simulink model "ROV_REG_SIM"  (R2014b)
settings: Solver=ode45  StartTime=0.0  StopTime=110  RelTol=1e-3
values from neighbouring files (symbols this model uses):
  ADB = 0.5    [ROV_REG.m]
  DDB = 0.8    [ROV_REG.m]
  Mass = 17    [ROV_REG.m]
  PT = [0,0,0,0,cos(ThDir(1,5:8)) ... (first row only)    [ROV_REG.m]
  rhoDB = rho/1000    (= 1)    [ROV_REG.m]
undefined symbols (not defined in the file or in its folder): magnitude
libraries: dspindex x4, vrlib x3
settings Model: Creator=Hartvik  LastModifiedBy=Hartvik

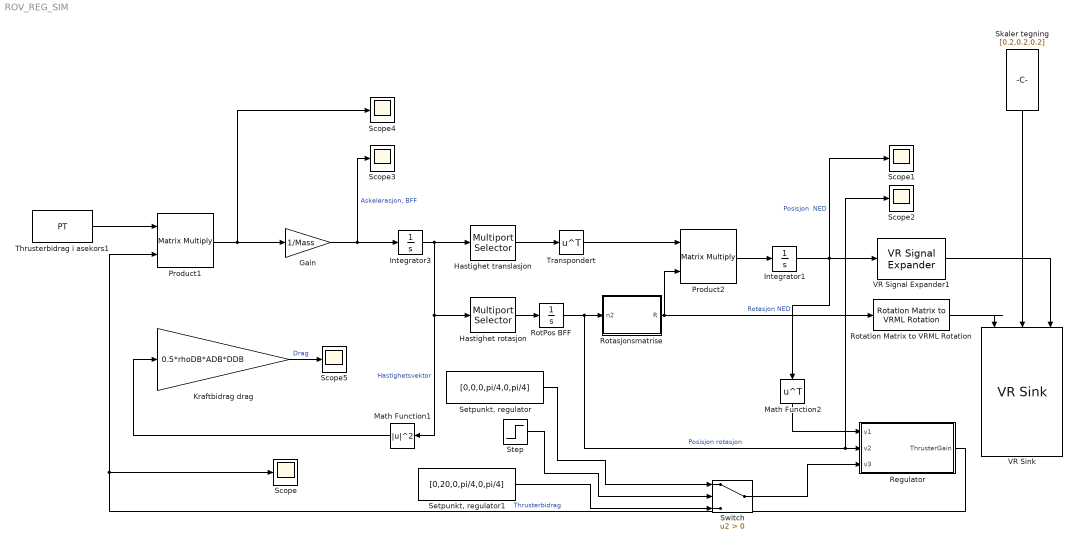
== system ROV_REG_SIM ==
  Gain : Gain  Gain=1/Mass
  Hastighet rotasjon : dspindex/Multiport Selector  rowsOrCols=Rows  idxCellArray={ 4:6}  idxErrMode=Clip Index
  Hastighet translasjon : dspindex/Multiport Selector  rowsOrCols=Rows  idxCellArray={ 1:3}  idxErrMode=Clip Index
  Integrator1 : Integrator
  Integrator3 : Integrator
  Kraftbidrag drag : Gain  Gain=0.5*rhoDB*ADB*DDB
  Math Function1 : Math  Operator=magnitude^2  SaturateOnIntegerOverflow=on
  Math Function2 : Math  Operator=transpose  SaturateOnIntegerOverflow=on
  Product1 : Product  Multiplication=Matrix(*)
  Product2 : Product  Multiplication=Matrix(*)
  Regulator : Subsystem  mask{Kd_rot=60, Kd_trans=10, Kp_rot=6, Kp_trans=1}
  RotPos BFF : Integrator
  Rotasjonsmatrise : MATLAB Function  TreatAsAtomicUnit=on
  Rotation Matrix to VRML Rotation : vrlib/Utilities/Rotation Matrix to VRML Rotation  maxzero=1e-12
  Scope{,1..5} (6 alike) : Scope
      Scope settings: YMin=-0.005  YMax=0.004
      Scope1 settings: TimeRange=37.52499999999999  YMin=0  YMax=1.4
      Scope2 settings: TimeRange=37.52499999999999  YMin=0  YMax=1.4  SaveName=ScopeData2
      Scope3 settings: YMin=-0.1  YMax=0.2  SaveName=ScopeData3
      Scope4 settings: YMin=-1e+15  YMax=8e+14  SaveName=ScopeData4
      Scope5 settings: YMin=-30  YMax=30  SaveName=ScopeData5
  "Setpunkt, regulator" : Constant  Value=[0,0,0,pi/4,0,pi/4]
  "Setpunkt, regulator1" : Constant  Value=[0,20,0,pi/4,0,pi/4]
  Skaler tegning : Constant  Value=[0.2,0.2,0.2]
  Step : Step  Time=15  Before=1  After=-1  SampleTime=0
  Switch : Switch  Criteria=u2 > Threshold
  Thrusterbidrag i asekors1 : Constant  Value=PT
  Transpondert : Math  Operator=transpose  SaturateOnIntegerOverflow=on
  VR Signal Expander1 : vrlib/VR Signal Expander  outwidth=3  outidx=[1,2,3]
  VR Sink : vrlib/VR Sink  InstantiateOnLoad=on  SampleTime=0.1  ViewEnable=on  RemoteChange=off  RemoteView=off  FieldsWritten=AUV.rotation.4.1.1.double#AUV.scale.3.1.1.double#AUV.translation.3.1.1.double  WorldFileName=D:\Dropbox\UISS-03-ROV\Elektro\Regulering\Simulink3D\AUV_emptyshell.wrl  WorldDescription=AUV_emptyshell  AutoView=off  VideoDimensions=[]  AllowVariableSize=off  FigureProperties="{'Position', 'Name', 'Viewpoint', 'CameraBound', 'CameraDirection', 'CameraPosition', 'CameraUpVector', 'ZoomFactor', 'Antialiasing', 'Headlight', 'Lighting', 'NavPanel', 'Sound', 'StatusBar', 'Stereo3D', 'Stereo3DCameraOffset', 'Stereo3DHIT', 'ToolBar', 'Textures', 'Transparency', 'Triad', 'Wireframe', 'NavZones', 'NavMode', 'NavSpeed', 'CaptureFileFormat', 'CaptureFileName', 'Record2DCompressMethod', 'Record2DCompressQuality', 'Record2D', 'Record2DFileName', 'Record2DFPS'; [5.0000000000000000e+00   9.2000000000000000e+01   5.7600000000000000e+02   3.8000000000000000e+02], 'AUV_emptyshell', 'Front', 'on', [0.0000000000000000e+00   0.0000000000000000e+00  -1.0000000000000000e+00], [0.0000000000000000e+00   0.0000000000000000e+00   0.0000000000000000e+00], [0.0000000000000000e+00   1.0000000000000000e+00   0.0000000000000000e+00], [1.0000000000000000e+00], 'on', 'on', 'on', 'halfbar', 'on', 'on', 'off', [1.0000000149011612e-01], [0.0000000000000000e+00], 'on', 'on', 'on', 'none', 'off', 'off', 'examine', 'normal', 'tif', '%f_anim_%n.tif', 'auto', [7.5000000000000000e+01], 'off', '%f_anim_%n.avi', 'auto'}"
  wires:
  Gain/1 -> Integrator3/1, Scope3/1  "Askelerasjon, BFF"
  Thrusterbidrag i asekors1/1 -> Product1/1
  Hastighet translasjon/1 -> Transpondert/1
  Transpondert/1 -> Product2/1
  Rotasjonsmatrise/1(R) -> Rotation Matrix to VRML Rotation/1, Product2/2  "Rotasjon NED"
  Regulator/1(ThrusterGain) -> Product1/2, Scope/1  "Thrusterbidrag"
  RotPos BFF/1 -> Regulator/2(v2), Scope2/1, Rotasjonsmatrise/1(n2)  "Posisjon rotasjon"
  Hastighet rotasjon/1 -> RotPos BFF/1
  Integrator1/1 -> VR Signal Expander1/1, Scope1/1, Math Function2/1  "Posisjon  NED"
  Integrator3/1 -> Math Function1/1, Hastighet rotasjon/1, Hastighet translasjon/1  "Hastighetsvektor"
  Math Function1/1 -> Kraftbidrag drag/1
  Kraftbidrag drag/1 -> Scope5/1  "Drag"
  Product1/1 -> Gain/1, Scope4/1
  Product2/1 -> Integrator1/1
  Math Function2/1 -> Regulator/1(v1)
  "Setpunkt, regulator1"/1 -> Switch/3
  Step/1 -> Switch/2
  Rotation Matrix to VRML Rotation/1 -> VR Sink/1
  VR Signal Expander1/1 -> VR Sink/3
  Skaler tegning/1 -> VR Sink/2
  "Setpunkt, regulator"/1 -> Switch/1
  Switch/1 -> Regulator/3(v3)

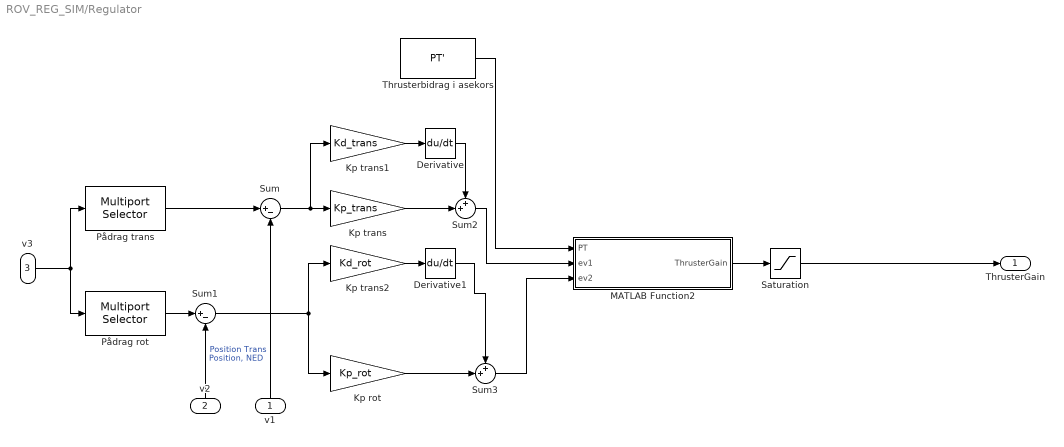
== system ROV_REG_SIM/Regulator ==
  v1 : Inport
  v2 : Inport  Port=2
  v3 : Inport  Port=3
  Derivative : Derivative
  Derivative1 : Derivative
  Kp rot : Gain  Gain=Kp_rot
  Kp trans : Gain  Gain=Kp_trans
  Kp trans1 : Gain  Gain=Kd_trans
  Kp trans2 : Gain  Gain=Kd_rot
  MATLAB Function2 : MATLAB Function  TreatAsAtomicUnit=on
  Pådrag rot : dspindex/Multiport Selector  rowsOrCols=Rows  idxCellArray={ 4:6}  idxErrMode=Clip Index
  Pådrag trans : dspindex/Multiport Selector  rowsOrCols=Rows  idxCellArray={ 1:3}  idxErrMode=Clip Index
  Saturation : Saturate  UpperLimit=20  LowerLimit=-20
  Sum : Sum  Inputs=|+-
  Sum1 : Sum  Inputs=|+-
  Sum2 : Sum  Inputs=++|
  Sum3 : Sum  Inputs=++|
  Thrusterbidrag i asekors : Constant  Value=PT'
  ThrusterGain : Outport
  wires:
  Thrusterbidrag i asekors/1 -> MATLAB Function2/1(PT)
  v3/1 -> Pådrag trans/1, Pådrag rot/1
  Pådrag trans/1 -> Sum/1
  v1/1 -> Sum/2  "Position Trans"
  MATLAB Function2/1(ThrusterGain) -> Saturation/1
  Pådrag rot/1 -> Sum1/1
  v2/1 -> Sum1/2  "Position, NED"
  Sum/1 -> Kp trans1/1, Kp trans/1
  Kp trans1/1 -> Derivative/1
  Kp trans/1 -> Sum2/2
  Sum1/1 -> Kp trans2/1, Kp rot/1
  Kp trans2/1 -> Derivative1/1
  Kp rot/1 -> Sum3/2
  Sum3/1 -> MATLAB Function2/3(ev2)
  Sum2/1 -> MATLAB Function2/2(ev1)
  Saturation/1 -> ThrusterGain/1
  Derivative1/1 -> Sum3/1
  Derivative/1 -> Sum2/1

== matlab function ROV_REG_SIM/Rotasjonsmatrise ==
  data: n2 input; R output
function R = fcn(n2)

R = [cos(n2(3))*cos(n2(2))  , -sin(n2(3))*cos(n2(1)) + cos(n2(3))*sin(n2(2))*sin(n2(1)) ,  sin(n2(3))*sin(n2(1)) + cos(n2(3))*sin(n2(2))*cos(n2(1))
     sin(n2(3))*cos(n2(2))  ,  cos(n2(3))*cos(n2(1)) + sin(n2(1))*sin(n2(2))*sin(n2(3)) , -cos(n2(3))*sin(n2(1)) + sin(n2(2))*sin(n2(3))*cos(n2(1))
               -sin(n2(2))  ,                                     cos(n2(2))*sin(n2(1)) , cos(n2(2))*cos(n2(1))
    ];

== matlab function ROV_REG_SIM/Regulator/MATLAB Function2 ==
  data: PT input; ThrusterGain output; ev1 input; ev2 input
function ThrusterGain = fcn(PT,ev1,ev2)
ThrusterGain = PT * [ev1;ev2];
